simulink model "electroMagnetModelStateSpace"  (R2016b)
settings: Solver=ode45  StartTime=0.0  StopTime=5  MaxStep=0.01  RelTol=1e-3  EnableMultiTasking=on
undefined symbols (not defined in the file): Ax, Bx, Cx, Dx, u_0, x_0
settings Model: Creator=dimpa  LastModifiedBy=Thomas
settings DataIOCC: LimitDataPoints=on  SaveFormat=Array
settings OptimizationCC: LifeSpan=inf
settings DebuggingCC: SolverPrmCheckMsg=warning  SFUnexpectedBacktrackingDiag=warning  SFNoUnconditionalDefaultTransitionDiag=warning  SFExecutionAtInitializationDiag=none
settings HardwareCC: ProdBitPerPointer=32  ProdBitPerSizeT=32  ProdBitPerPtrDiffT=32  ProdLargestAtomicFloat=None  ProdIntDivRoundTo=Undefined  ProdEndianess=Unspecified  ProdWordSize=32  ProdHWDeviceType=32-bit Generic
settings ModelReferenceCC: PropagateSignalLabelsOutOfModel=off
settings GRTTargetCC: TargetLangStandard=C89/C90 (ANSI)  GeneratePreprocessorConditionals=Disable all
settings ConfigComp: CovMetricSettings=dw  CovHtmlReporting=on  CovSaveCumulativeToWorkspaceVar=on  CovSaveSingleToWorkspaceVar=on  CovExternalEMLEnable=off  CovSFcnEnable=off

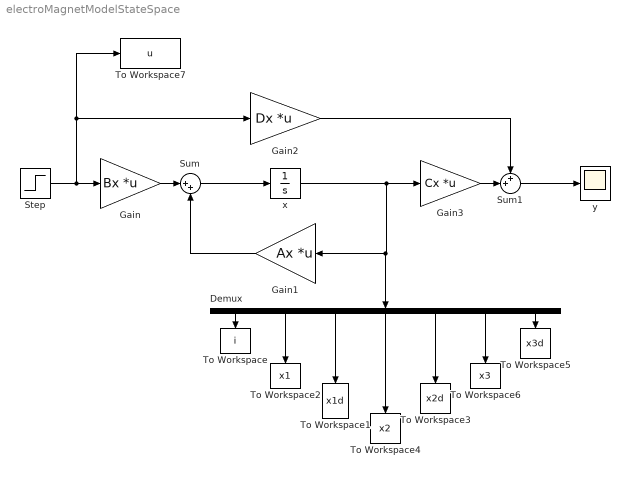
== system electroMagnetModelStateSpace ==
  Demux : Demux  Outputs=7
  Gain : Gain  Gain=Bx  Multiplication=Matrix(K*u) (u vector)
  Gain1 : Gain  Gain=Ax  Multiplication=Matrix(K*u) (u vector)
  Gain2 : Gain  Gain=Dx  Multiplication=Matrix(K*u) (u vector)
  Gain3 : Gain  Gain=Cx  Multiplication=Matrix(K*u) (u vector)
  Step : Step  After=u_0  SampleTime=0
  Sum : Sum  Inputs=|++
  Sum1 : Sum  Inputs=++|
  To Workspace : ToWorkspace  VariableName=i  SaveFormat=Structure With Time  SampleTime=-1
  To Workspace1 : ToWorkspace  VariableName=x1d  SaveFormat=Structure With Time  SampleTime=-1
  To Workspace2 : ToWorkspace  VariableName=x1  SaveFormat=Structure With Time  SampleTime=-1
  To Workspace3 : ToWorkspace  VariableName=x2d  SaveFormat=Structure With Time  SampleTime=-1
  To Workspace4 : ToWorkspace  VariableName=x2  SaveFormat=Structure With Time  SampleTime=-1
  To Workspace5 : ToWorkspace  VariableName=x3d  SaveFormat=Structure With Time  SampleTime=-1
  To Workspace6 : ToWorkspace  VariableName=x3  SaveFormat=Structure With Time  SampleTime=-1
  To Workspace7 : ToWorkspace  VariableName=u  SaveFormat=Structure With Time  SampleTime=-1
  x : Integrator  InitialCondition=x_0
  y : Scope
  wires:
  x/1 -> Demux/1, Gain1/1, Gain3/1
  Step/1 -> To Workspace7/1, Gain2/1, Gain/1
  Sum/1 -> x/1
  Gain/1 -> Sum/1
  Gain1/1 -> Sum/2
  Gain2/1 -> Sum1/1
  Gain3/1 -> Sum1/2
  Sum1/1 -> y/1
  Demux/1 -> To Workspace/1
  Demux/2 -> To Workspace2/1
  Demux/3 -> To Workspace1/1
  Demux/4 -> To Workspace4/1
  Demux/5 -> To Workspace3/1
  Demux/6 -> To Workspace6/1
  Demux/7 -> To Workspace5/1
